simulink model "model_depillis_2016"  (R2016b)
settings: Solver=FixedStepAuto  StartTime=0  StopTime=150  FixedStep=0.1  RelTol=1e-3
settings Model: Creator=bsolv  LastModifiedBy=Jay

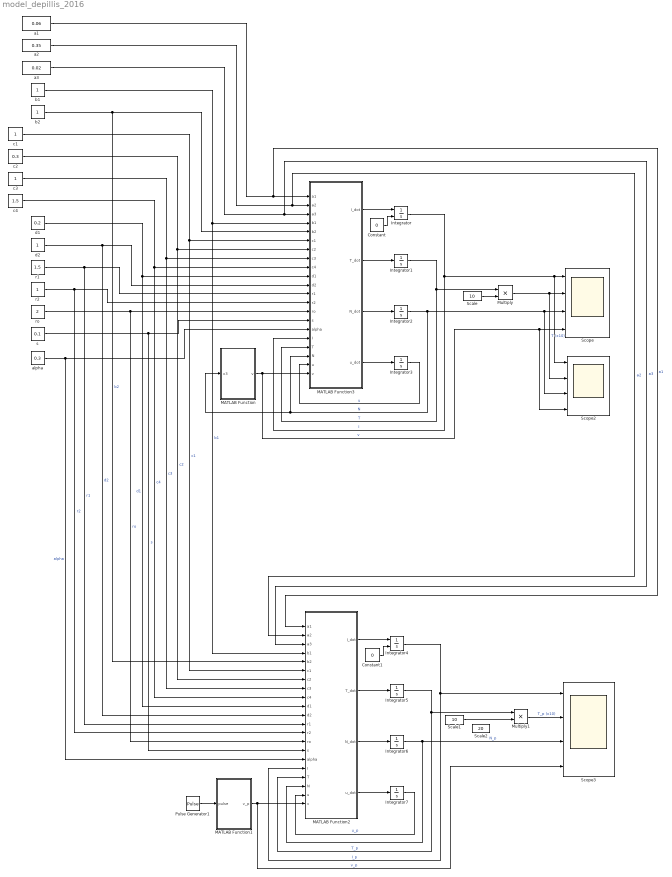
== system model_depillis_2016 ==
  Constant : Constant  Value=0
  Constant1 : Constant  Value=0
  Integrator : Integrator  InitialConditionSource=external
  Integrator1 : Integrator  InitialCondition=10^-5
  Integrator2 : Integrator  InitialCondition=1
  Integrator3 : Integrator
  Integrator4 : Integrator  InitialConditionSource=external
  Integrator5 : Integrator  InitialCondition=10^-5
  Integrator6 : Integrator  InitialCondition=1
  Integrator7 : Integrator
  MATLAB Function : MATLAB Function  TreatAsAtomicUnit=on
  MATLAB Function1 : MATLAB Function  TreatAsAtomicUnit=on
  MATLAB Function2 : MATLAB Function  TreatAsAtomicUnit=on
  MATLAB Function3 : MATLAB Function  TreatAsAtomicUnit=on
  Multiply : Product
  Multiply1 : Product
  Pulse Generator1 : DiscretePulseGenerator  Period=20
  Scale : Constant  Value=10
  Scale1 : Constant  Value=10
  Scale2 : Constant  Value=20
  Scope : Scope  NumInputPorts=4
  Scope2 : Scope  NumInputPorts=4
  Scope3 : Scope  NumInputPorts=4
  a1 : Constant  Value=0.06
  a2 : Constant  Value=0.35
  a3 : Constant  Value=0.02
  alpha : Constant  Value=0.3
  b1 : Constant
  b2 : Constant
  c1 : Constant
  c2 : Constant  Value=0.3
  c3 : Constant
  c4 : Constant  Value=1.5
  d1 : Constant  Value=0.2
  d2 : Constant
  r1 : Constant  Value=1.5
  r2 : Constant
  ro : Constant  Value=2
  s : Constant  Value=0.1
  wires:
  a1/1 -> MATLAB Function2/1(a1), MATLAB Function3/1(a1)  "a1"
  a2/1 -> MATLAB Function2/2(a2), MATLAB Function3/2(a2)  "a2"
  a3/1 -> MATLAB Function2/3(a3), MATLAB Function3/3(a3)  "a3"
  c1/1 -> MATLAB Function2/6(c1), MATLAB Function3/6(c1)  "c1"
  c2/1 -> MATLAB Function2/7(c2), MATLAB Function3/7(c2)  "c2"
  c3/1 -> MATLAB Function2/8(c3), MATLAB Function3/8(c3)  "c3"
  c4/1 -> MATLAB Function2/9(c4), MATLAB Function3/9(c4)  "c4"
  MATLAB Function3/1(I_dot) -> Integrator/1
  MATLAB Function3/2(T_dot) -> Integrator1/1
  MATLAB Function3/3(N_dot) -> Integrator2/1
  MATLAB Function3/4(u_dot) -> Integrator3/1
  Integrator/1 -> MATLAB Function3/17(I), Scope2/1, Scope/1  "I"
  Integrator1/1 -> Multiply/1, MATLAB Function3/18(T)  "T"
  Integrator2/1 -> MATLAB Function3/19(N), MATLAB Function/1(x3), Scope2/3, Scope/3  "N"
  Integrator3/1 -> MATLAB Function3/20(u)  "u"
  MATLAB Function/1(v) -> Scope2/4, Scope/4, MATLAB Function3/21(v)  "v"
  Scale/1 -> Multiply/2
  Multiply/1 -> Scope2/2, Scope/2  "T (x10)"
  Constant/1 -> Integrator/2
  alpha/1 -> MATLAB Function2/16(alpha), MATLAB Function3/16(alpha)  "alpha"
  MATLAB Function2/3(N_dot) -> Integrator6/1
  MATLAB Function2/1(I_dot) -> Integrator4/1
  Constant1/1 -> Integrator4/2
  Multiply1/1 -> Scope3/2  "T_p (x10)"
  MATLAB Function1/1(v_p) -> Scope3/4, MATLAB Function2/21(v)  "v_p"
  Integrator7/1 -> MATLAB Function2/20(u)  "u_p"
  r2/1 -> MATLAB Function2/13(r2), MATLAB Function3/13(r2)  "r2"
  d2/1 -> MATLAB Function2/11(d2), MATLAB Function3/11(d2)  "d2"
  d1/1 -> MATLAB Function2/10(d1), MATLAB Function3/10(d1)  "d1"
  s/1 -> MATLAB Function2/15(s), MATLAB Function3/15(s)  "s"
  Integrator6/1 -> Scope3/3, MATLAB Function2/19(N)  "N_p"
  Integrator5/1 -> MATLAB Function2/18(T), Multiply1/1  "T_p"
  Integrator4/1 -> MATLAB Function2/17(I), Scope3/1  "I_p"
  MATLAB Function2/2(T_dot) -> Integrator5/1
  b2/1 -> MATLAB Function2/5(b2), MATLAB Function3/5(b2)  "b2"
  ro/1 -> MATLAB Function2/14(ro), MATLAB Function3/14(ro)  "ro"
  r1/1 -> MATLAB Function2/12(r1), MATLAB Function3/12(r1)  "r1"
  b1/1 -> MATLAB Function2/4(b1), MATLAB Function3/4(b1)  "b1"
  MATLAB Function2/4(u_dot) -> Integrator7/1
  Pulse Generator1/1 -> MATLAB Function1/1(pulse)
  Scale1/1 -> Multiply1/2

== matlab function model_depillis_2016/MATLAB Function1 ==
  data: pulse input; v_p output
function v_p = drug(pulse)
% 
%     if x3 < 0.92
%         v = 1;
%     else
%         v = 0;        
%     end
%     
    v_p=0;
    if pulse
        v_p=1;
    end

== matlab function model_depillis_2016/MATLAB Function ==
  data: x3 input; v output
function v = drug(x3)

    if x3 < 0.95 %0.955
        
        v = 1;
    else
        v = 0;        
    end
    
%     v=0;
%     if pulse
%         v=1;
%     end

== matlab function model_depillis_2016/MATLAB Function2 ==
  data: a1 input; I_dot output; a2 input; a3 input; b1 input; b2 input; c1 input; c2 input; c3 input; c4 input; d1 input; d2 input; r1 input; r2 input; ro input; s input; alpha input; I input; T input; N input; u input; v input; T_dot output; N_dot output; u_dot output
function [I_dot, T_dot, N_dot, u_dot] = Derivatives(a1, a2, a3, b1, b2, c1, c2, c3, c4, d1, d2, r1, r2, ro, s, alpha, I, T, N, u, v)
    % I,T,N,u - x1,x2,x3,x4
    
    %% Initial Conditions
%     Io = s/d1;
%     To = 10^-5;
%     No = 1;
%     An initial tumor population of 10^-5 normalized units is equivalent to 10^6 tumor cells;
    %% Reduced Immune response
%     ro = 1.5;
%     c1 = 0.6;
%     c2 = 0.5;
%     c3 = 0.1;
%     r1 = 30;
    
    %% Increased Immune response
%     ro = 2.0;
    
    %%

    I_dot = s + ro*I*T/(alpha+T) - c1*I*T - d1*I - a1*(1 -exp(-u))*I;
    T_dot = r1*T*(1-b1*T) - c2*I*T - c3*T*N - a2*(1 -exp(-u))*T;
    N_dot = r2*N*(1-b2*N) - c4*T*N - a3*(1 -exp(-u))*N;
    u_dot = v - d2*u;
    
    %% Nondimensional
%     x1 = I;
%     x2 = T;
%     x3 = N;
%     x4 = u;
%     p1 = 
%     p2 = 
%     p3 = 
%     p4 = 
    
%     p1_dot = -p1*( ro*x2/(alpha +x2) -c1*x2 -d1 -a1*(1-exp(-x4))) +p2*c2*x2;
%     p2_dot = -p1*( ro*alpha*x1/( alpha +x2)^2 -c1*x1) -p2*( r1 -2*r1*b1*x2 -c2*x1 -c3*x3 -a2*(1-exp(-x4))) +p3*c4*x3;
%     p3_dot = p2*c3*x3 -p3*( r2 -2*r2*x3^2 -c4*x2 -a3*(1-exp(-x4))) -eta;
%     p4_dot = -exp(-x4)*( a1*p1*x1 +a2*p2*x2 +a3*p3*x3);

end

== matlab function model_depillis_2016/MATLAB Function3 ==
  data: a1 input; I_dot output; a2 input; a3 input; b1 input; b2 input; c1 input; c2 input; c3 input; c4 input; d1 input; d2 input; r1 input; r2 input; ro input; s input; alpha input; I input; T input; N input; u input; v input; T_dot output; N_dot output; u_dot output
function [I_dot, T_dot, N_dot, u_dot] = Derivatives(a1, a2, a3, b1, b2, c1, c2, c3, c4, d1, d2, r1, r2, ro, s, alpha, I, T, N, u, v)
    % I,T,N,u - x1,x2,x3,x4
    
    %% Initial Conditions
%     Io = s/d1;
%     To = 10^-5;
%     No = 1;
%     An initial tumor population of 10^-5 normalized units is equivalent to 10^6 tumor cells;
    %% Reduced Immune response
%     ro = 1.5;
%     c1 = 0.6;
%     c2 = 0.5;
%     c3 = 0.1;
%     r1 = 30;
    
    %% Increased Immune response
%     ro = 2.0;
    
    %%

    I_dot = s + ro*I*T/(alpha+T) - c1*I*T - d1*I - a1*(1 -exp(-u))*I;
    T_dot = r1*T*(1-b1*T) - c2*I*T - c3*T*N - a2*(1 -exp(-u))*T;
    N_dot = r2*N*(1-b2*N) - c4*T*N - a3*(1 -exp(-u))*N;
    u_dot = v - d2*u;
    
    %% Nondimensional
%     x1 = I;
%     x2 = T;
%     x3 = N;
%     x4 = u;
%     p1 = 
%     p2 = 
%     p3 = 
%     p4 = 
    
%     p1_dot = -p1*( ro*x2/(alpha +x2) -c1*x2 -d1 -a1*(1-exp(-x4))) +p2*c2*x2;
%     p2_dot = -p1*( ro*alpha*x1/( alpha +x2)^2 -c1*x1) -p2*( r1 -2*r1*b1*x2 -c2*x1 -c3*x3 -a2*(1-exp(-x4))) +p3*c4*x3;
%     p3_dot = p2*c3*x3 -p3*( r2 -2*r2*x3^2 -c4*x2 -a3*(1-exp(-x4))) -eta;
%     p4_dot = -exp(-x4)*( a1*p1*x1 +a2*p2*x2 +a3*p3*x3);

end
